simulink model "ask2"  (R2016a)
settings: Solver=VariableStepAuto  StartTime=0.0  StopTime=0.5  RelTol=1e-3
values from neighbouring files (symbols this model uses):
  kb = 26.3    [ex1.m]
  kbp = 1    [ex1.m]
  ki = 193*kbp    (= 193)    [ex1.m]
libraries: simulink x1
settings Model: Creator=JIM  LastModifiedBy=JIM

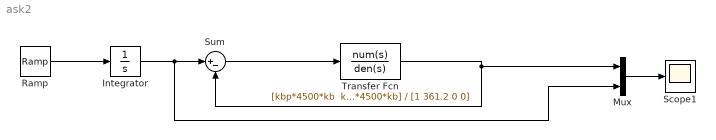
== system ask2 ==
  Integrator : Integrator
  Mux : Mux  Inputs=2
  Ramp : simulink/Sources/Ramp  slope=1  start=0  X0=0
  Scope1 : Scope
  Sum : Sum  Inputs=|+-
  Transfer Fcn : TransferFcn  Numerator="[kbp*4500*kb  ki*4500*kb]"  Denominator=[1 361.2 0 0]
  wires:
  Transfer Fcn/1 -> Sum/2, Mux/1
  Sum/1 -> Transfer Fcn/1
  Integrator/1 -> Mux/2, Sum/1
  Mux/1 -> Scope1/1
  Ramp/1 -> Integrator/1
